simulink model "space_actuator_model"  (R2024b)
settings: Solver=ode23  StartTime=0.0  StopTime=5  RelTol=1e-3
settings Model: Creator=Ahsile  LastModifiedBy=Ahsile

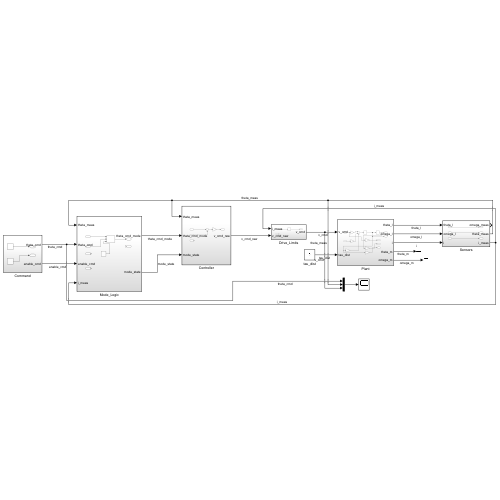
[thumbnail: Simulink's stored preview of the top-level diagram]
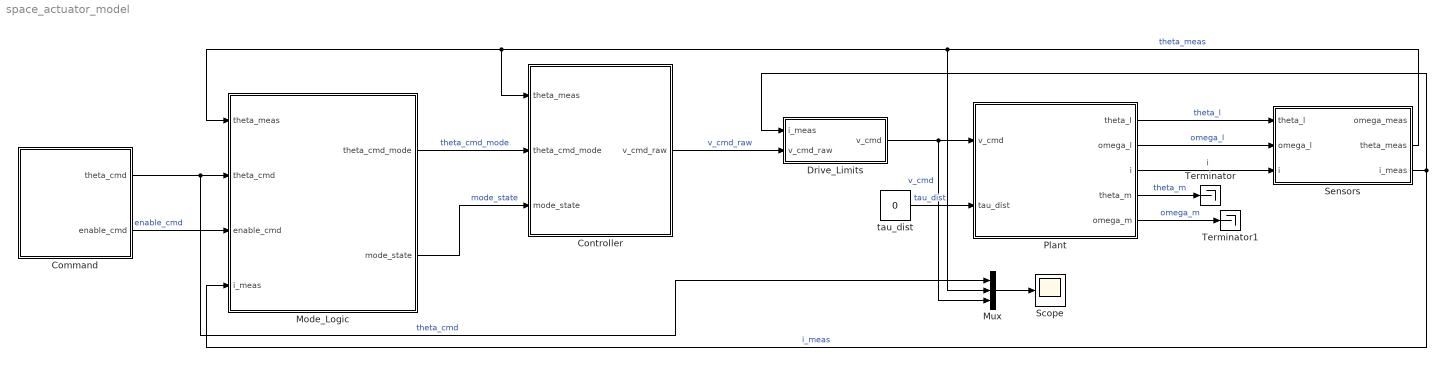
== system space_actuator_model ==
  Command : Subsystem
  Controller : Subsystem
  Drive_Limits : Subsystem
  Mode_Logic : Subsystem
  Mux : Mux  Inputs=3
  Plant : Subsystem
  Scope : Scope
  Sensors : Subsystem
  Terminator : Terminator
  Terminator1 : Terminator
  tau_dist : Constant  Value=0
  wires:
  Mode_Logic/1(theta_cmd_mode) -> Controller/2(theta_cmd_mode)  "theta_cmd_mode"
  Controller/1(v_cmd_raw) -> Drive_Limits/2(v_cmd_raw)  "v_cmd_raw"
  Drive_Limits/1(v_cmd) -> Plant/1(v_cmd), Mux/3  "v_cmd"
  Plant/1(theta_l) -> Sensors/1(theta_l)  "theta_l"
  Sensors/2(theta_meas) -> Mux/2, Controller/1(theta_meas), Mode_Logic/1(theta_meas)  "theta_meas"
  Command/1(theta_cmd) -> Mux/1, Mode_Logic/2(theta_cmd)  "theta_cmd"
  Command/2(enable_cmd) -> Mode_Logic/3(enable_cmd)  "enable_cmd"
  Mode_Logic/2(mode_state) -> Controller/3(mode_state)  "mode_state"
  Sensors/3(i_meas) -> Drive_Limits/1(i_meas), Mode_Logic/4(i_meas)  "i_meas"
  Plant/2(omega_l) -> Sensors/2(omega_l)  "omega_l"
  Plant/3(i) -> Sensors/3(i)  "i"
  tau_dist/1 -> Plant/2(tau_dist)  "tau_dist"
  Plant/4(theta_m) -> Terminator/1  "theta_m"
  Plant/5(omega_m) -> Terminator1/1  "omega_m"
  Mux/1 -> Scope/1

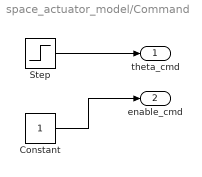
== system space_actuator_model/Command ==
  Constant : Constant
  Step : Step  Time=.5  After=.2  SampleTime=0
  theta_cmd : Outport
  enable_cmd : Outport  Port=2
  wires:
  Step/1 -> theta_cmd/1
  Constant/1 -> enable_cmd/1

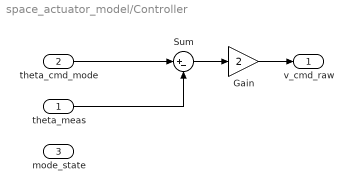
== system space_actuator_model/Controller ==
  theta_meas : Inport
  theta_cmd_mode : Inport  Port=2
  mode_state : Inport  Port=3
  Gain : Gain  Gain=2
  Sum : Sum  Inputs=|+-
  v_cmd_raw : Outport
  wires:
  theta_cmd_mode/1 -> Sum/1
  theta_meas/1 -> Sum/2
  Sum/1 -> Gain/1
  Gain/1 -> v_cmd_raw/1

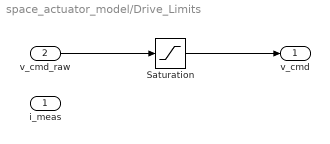
== system space_actuator_model/Drive_Limits ==
  i_meas : Inport
  v_cmd_raw : Inport  Port=2
  Saturation : Saturate  UpperLimit=24  LowerLimit=-24
  v_cmd : Outport
  wires:
  v_cmd_raw/1 -> Saturation/1
  Saturation/1 -> v_cmd/1

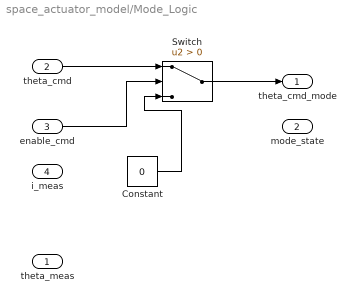
== system space_actuator_model/Mode_Logic ==
  theta_meas : Inport
  theta_cmd : Inport  Port=2
  enable_cmd : Inport  Port=3
  i_meas : Inport  Port=4
  Constant : Constant  Value=0
  Switch : Switch  Criteria=u2 > Threshold  SaturateOnIntegerOverflow=off  InputSameDT=off
  theta_cmd_mode : Outport
  mode_state : Outport  Port=2
  wires:
  theta_cmd/1 -> Switch/1
  Constant/1 -> Switch/3
  enable_cmd/1 -> Switch/2
  Switch/1 -> theta_cmd_mode/1

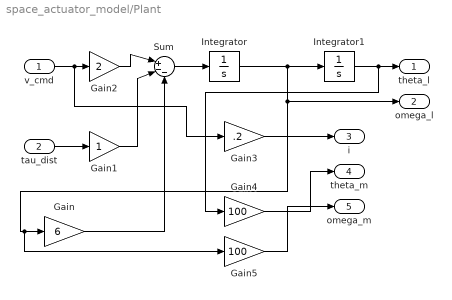
== system space_actuator_model/Plant ==
  v_cmd : Inport
  tau_dist : Inport  Port=2
  Gain : Gain  Gain=6
  Gain1 : Gain
  Gain2 : Gain  Gain=2
  Gain3 : Gain  Gain=.2
  Gain4 : Gain  Gain=100
  Gain5 : Gain  Gain=100
  Integrator : Integrator
  Integrator1 : Integrator
  Sum : Sum  Inputs=|+--
  theta_l : Outport
  omega_l : Outport  Port=2
  i : Outport  Port=3
  theta_m : Outport  Port=4
  omega_m : Outport  Port=5
  wires:
  Integrator1/1 -> Gain4/1, theta_l/1
  v_cmd/1 -> Gain3/1, Gain2/1
  Gain2/1 -> Sum/1
  tau_dist/1 -> Gain1/1
  Gain1/1 -> Sum/2
  Sum/1 -> Integrator/1
  Integrator/1 -> Integrator1/1, omega_l/1, Gain5/1, Gain/1
  Gain/1 -> Sum/3
  Gain3/1 -> i/1
  Gain4/1 -> theta_m/1
  Gain5/1 -> omega_m/1

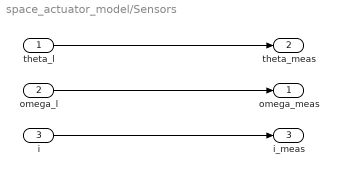
== system space_actuator_model/Sensors ==
  theta_l : Inport
  omega_l : Inport  Port=2
  i : Inport  Port=3
  omega_meas : Outport
  theta_meas : Outport  Port=2
  i_meas : Outport  Port=3
  wires:
  theta_l/1 -> theta_meas/1
  omega_l/1 -> omega_meas/1
  i/1 -> i_meas/1
